simulink model "Encryption_Model"  (R2021a)
settings: Solver=VariableStepAuto  StartTime=0.0  StopTime=10.0  RelTol=1e-3
settings Model: Creator=a080754  LastModifiedBy=a080754

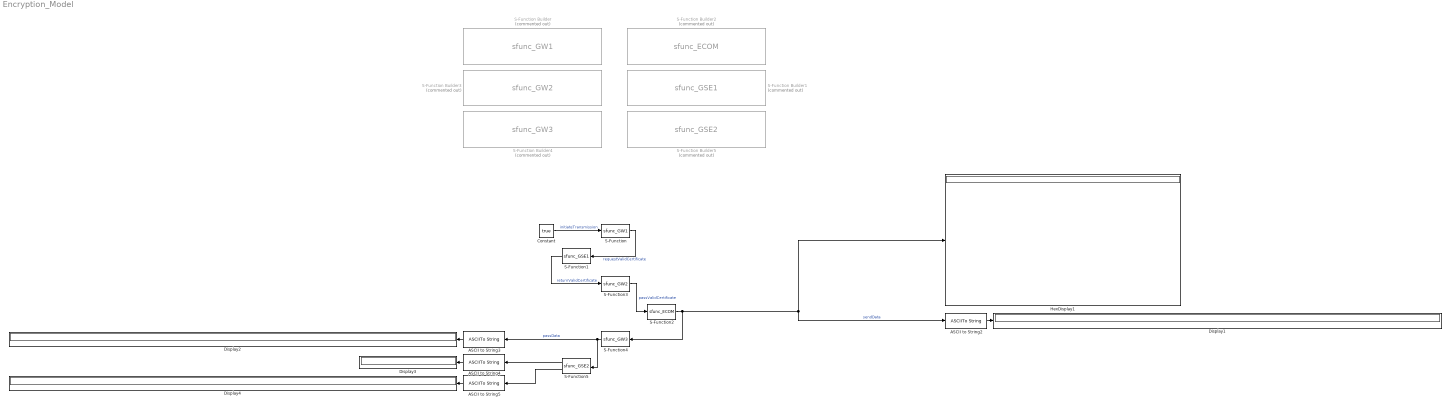
== system Encryption_Model ==
  ASCII to String{2..5} (4 alike) : ASCIIToString
  Constant : Constant  Value=true  OutDataTypeStr=boolean
  Display{1..4} (4 alike) : Display
  HexDisplay1 : Display
      settings: Format=hex (Stored Integer)
  S-Function : S-Function  FunctionName=sfunc_GW1  SFunctionDeploymentMode=off  EnableBusSupport=off
  S-Function Builder : S-Function  Commented=on  FunctionName=sfunc_GW1  SFunctionModules=sfunc_GW1_wrapper  SFunctionDeploymentMode=off  EnableBusSupport=off  mask(S-Function Builder){}
      mask help: Simulink:masks:SFunctionBuilder_MD
      mask init:
      | val = [[.9  0.75 0.75 1 1 .9 .9 1]',[1 1 0.75 0.75 .9 .9 1 .9]'];try , sys = get_param(gcb,'SfunBuilderFcnName');if isempty(sys), sys = get_param(gcb,'FunctionName'); end,catch, sys = get_param(gcb,'FunctionName'); end
      settings: CopyFcn=set_param(gcbh,'LinkStatus','none')  OpenFcn=sfunctionwizard(gcbh)
      mask Display: plot(val(:,1),val(:,2)),disp(sys),port_label('input',1,'gw_input_mid'),port_label('output',1,'gw_output')
  S-Function Builder1 : S-Function  Commented=on  FunctionName=sfunc_GSE1  SFunctionModules=sfunc_GSE1_wrapper  SFunctionDeploymentMode=off  EnableBusSupport=off  mask(S-Function Builder){}
      mask help: Simulink:masks:SFunctionBuilder_MD
      mask init: same as Encryption_Model/S-Function Builder
      settings: CopyFcn=set_param(gcbh,'LinkStatus','none')  OpenFcn=sfunctionwizard(gcbh)
      mask Display:
      | plot(val(:,1),val(:,2))
      | disp(sys)
      | port_label('input',1,'gse_input')
      | port_label('output',1,'gse_output_name')
  S-Function Builder2 : S-Function  Commented=on  FunctionName=sfunc_ECOM  SFunctionModules=sfunc_ECOM_wrapper  SFunctionDeploymentMode=off  EnableBusSupport=off  mask(S-Function Builder){}
      mask help: Simulink:masks:SFunctionBuilder_MD
      mask init: same as Encryption_Model/S-Function Builder
      settings: CopyFcn=set_param(gcbh,'LinkStatus','none')  OpenFcn=sfunctionwizard(gcbh)
      mask Display: plot(val(:,1),val(:,2)),disp(sys),port_label('input',1,'ecom_input_name'),port_label('output',1,'ecom_output')
  S-Function Builder3 : S-Function  Commented=on  FunctionName=sfunc_GW2  SFunctionModules=sfunc_GW2_wrapper  SFunctionDeploymentMode=off  EnableBusSupport=off  mask(S-Function Builder){}
      mask help: Simulink:masks:SFunctionBuilder_MD
      mask init: same as Encryption_Model/S-Function Builder
      settings: CopyFcn=set_param(gcbh,'LinkStatus','none')  OpenFcn=sfunctionwizard(gcbh)
      mask Display: plot(val(:,1),val(:,2)),disp(sys),port_label('input',1,'gw_input_name'),port_label('output',1,'gw_output_name')
  S-Function Builder4 : S-Function  Commented=on  FunctionName=sfunc_GW3  SFunctionModules=sfunc_GW3_wrapper  SFunctionDeploymentMode=off  EnableBusSupport=off  mask(S-Function Builder){}
      mask help: Simulink:masks:SFunctionBuilder_MD
      mask init: same as Encryption_Model/S-Function Builder
      settings: CopyFcn=set_param(gcbh,'LinkStatus','none')  OpenFcn=sfunctionwizard(gcbh)
      mask Display:
      | plot(val(:,1),val(:,2))
      | disp(sys)
      | port_label('input',1,'gw_input')
      | port_label('output',1,'gw_output')
  S-Function Builder5 : S-Function  Commented=on  FunctionName=sfunc_GSE2  SFunctionModules=sfunc_GSE2_wrapper  SFunctionDeploymentMode=off  EnableBusSupport=off  mask(S-Function Builder){}
      mask help: Simulink:masks:SFunctionBuilder_MD
      mask init: same as Encryption_Model/S-Function Builder
      settings: CopyFcn=set_param(gcbh,'LinkStatus','none')  OpenFcn=sfunctionwizard(gcbh)
      mask Display:
      | plot(val(:,1),val(:,2))
      | disp(sys)
      | port_label('input',1,'gse_input')
      | port_label('output',1,'gse_output_plain')
      | port_label('output',2,'gse_output_cipher')
  S-Function1 : S-Function  FunctionName=sfunc_GSE1  SFunctionDeploymentMode=off  EnableBusSupport=off
  S-Function2 : S-Function  FunctionName=sfunc_ECOM  SFunctionDeploymentMode=off  EnableBusSupport=off
  S-Function3 : S-Function  FunctionName=sfunc_GW2  SFunctionDeploymentMode=off  EnableBusSupport=off
  S-Function4 : S-Function  FunctionName=sfunc_GW3  SFunctionDeploymentMode=off  EnableBusSupport=off
  S-Function5 : S-Function  FunctionName=sfunc_GSE2  SFunctionDeploymentMode=off  EnableBusSupport=off
  wires:
  Constant/1 -> S-Function/1  "initiateTransmission"
  S-Function/1 -> S-Function1/1  "requestValidCertificate"
  S-Function1/1 -> S-Function3/1  "returnValidCertificate"
  S-Function3/1 -> S-Function2/1  "passValidCertificate"
  S-Function2/1 -> ASCII to String2/1, HexDisplay1/1, S-Function4/1  "sendData"
  ASCII to String2/1 -> Display1/1
  ASCII to String3/1 -> Display2/1
  ASCII to String4/1 -> Display3/1
  ASCII to String5/1 -> Display4/1
  S-Function5/1 -> ASCII to String4/1
  S-Function5/2 -> ASCII to String5/1
  S-Function4/1 -> ASCII to String3/1, S-Function5/1  "passData"
